simulink model "sampleModel244"  (R2021b)
settings: Solver=VariableStepAuto  StartTime=0.0  StopTime=10.0  RelTol=1e-3
undefined symbols (not defined in the file or in its folder): DiscIntNeverNeededParam
libraries: simulink x13, slpidlib x3
settings Model: Creator=user  LastModifiedBy=user

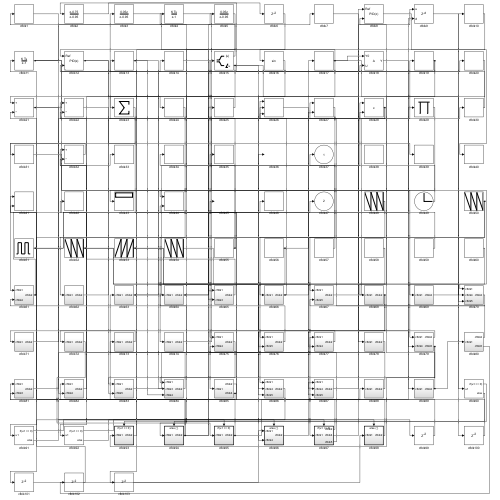
[thumbnail: Simulink's stored preview of the top-level diagram]
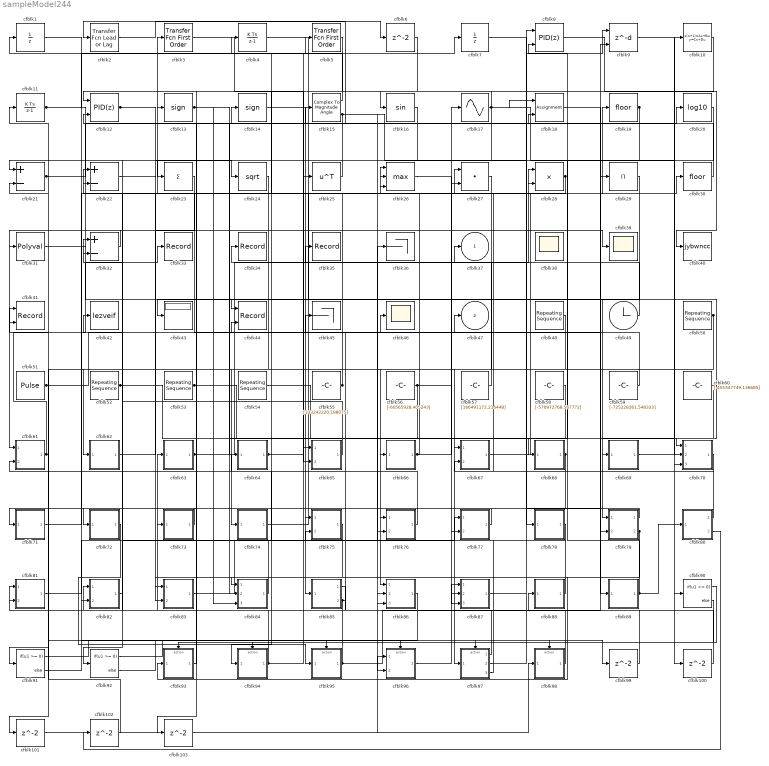
== system sampleModel244 ==
  cfblk1 : UnitDelay  HasFrameUpgradeWarning=on
  cfblk10 : DiscreteStateSpace
  cfblk{6,99..103} (6 alike) : Delay  SampleTime=1
  cfblk11 : DiscreteIntegrator  ICPrevOutput=DiscIntNeverNeededParam  ICPrevScaledInput=DiscIntNeverNeededParam
  cfblk12 : slpidlib/PID Controller (2DOF)  Controller=PID  Form=Parallel  TimeDomain=Discrete-time  UseExternalTs=off  SampleTime=1  IntegratorMethod=Forward Euler  FilterMethod=Forward Euler  ControllerParametersSource=internal  P=1  I=1  D=0  UseFilter=on  N=100  b=1  c=1  TunerSelectOption=Transfer Function Based (PID Tuner App)  InitialConditionSource=internal  InitialConditionForIntegrator=0  InitialConditionForFilter=0  DifferentiatorICPrevScaledInput=0  ExternalReset=none  TrackingMode=off  Kt=1  LimitOutput=off  SatLimitsSource=internal  UpperSaturationLimit=inf  LowerSaturationLimit=-inf  LinearizeAsGain=off  AntiWindupMode=none  Kb=1  POutMin=[]  POutMax=[]  IOutMin=[]  IOutMax=[]  DOutMin=[]  DOutMax=[]  NOutMin=[]  NOutMax=[]  bOutMin=[]  bOutMax=[]  cOutMin=[]  cOutMax=[]  SumOutMin=[]  SumOutMax=[]  SaturationOutMin=[]  SaturationOutMax=[]  PParamMin=[]  PParamMax=[]  IParamMin=[]  IParamMax=[]  DParamMin=[]  DParamMax=[]  NParamMin=[]  NParamMax=[]  bParamMin=[]  bParamMax=[]  cParamMin=[]  cParamMax=[]  KbParamMin=[]  KbParamMax=[]  KtParamMin=[]  KtParamMax=[]  KbOutMin=[]  KbOutMax=[]  KtOutMin=[]  KtOutMax=[]  IntegratorOutMin=[]  IntegratorOutMax=[]  FilterOutMin=[]  FilterOutMax=[]  SumI1OutMin=[]  SumI1OutMax=[]  SumI2OutMin=[]  SumI2OutMax=[]  SumI3OutMin=[]  SumI3OutMax=[]  SumI4OutMin=[]  SumI4OutMax=[]  SumDOutMin=[]  SumDOutMax=[]  Sum1OutMin=[]  Sum1OutMax=[]  Sum2OutMin=[]  Sum2OutMax=[]  Sum3OutMin=[]  Sum3OutMax=[]  DifferentiatorOutMin=[]  DifferentiatorOutMax=[]  FilterDiffOutCoefMin=[]  FilterDiffOutCoefMax=[]  ReciprocalOutMin=[]  ReciprocalOutMax=[]  SumDenOutMin=[]  SumDenOutMax=[]  SumNumOutMin=[]  SumNumOutMax=[]  DivideOutMin=[]  DivideOutMax=[]  UdiffTsProdOutMin=[]  UdiffTsProdOutMax=[]  NTsProdOutMin=[]  NTsProdOutMax=[]  UintegralTsProdOutMin=[]  UintegralTsProdOutMax=[]  UngainTsProdOutMin=[]  UngainTsProdOutMax=[]  IntegratorContinuousStateAttributes=''  IntegratorStateMustResolveToSignalObject=off  IntegratorRTWStateStorageClass=Auto  FilterContinuousStateAttributes=''  FilterStateMustResolveToSignalObject=off  FilterRTWStateStorageClass=Auto  ParallelPVariant=InternalParameters  IdealPVariant=Disabled  IVariant=InternalParameters  DVariant=InternalParameters  bVariant=InternalParameters  cVariant=InternalParameters  IntegratorVariant=Discrete  SatVariant=Disabled  AWVariant=Passthrough  PCopyVariant=Disabled  TRVariant=Disabled  FdbkBlocksVariant=Forward  IdealPFdbkVariant=Disabled  SatFdbkVariant=Disabled  DerivativeFilterVariant=ForwardEulerFilter  NVariant=InternalParameters  NCopyVariant=Disabled  FilterICVariant=InternalICsFilter  IntegratorICVariant=InternalICs  ExternalResetVariant=Disabled  TRSumVariant=Passthrough  SumFdbkVariant=Disabled  SumVariant=Sum_PID  TsampFilterVariant=InternalTs  TsampNgainVariant=Passthrough  TsampIntegralVariant=Passthrough  ExternalSaturationOutDataTypeStr=Inherit: Same as second input
      settings: SourceProductBaseCode=SL
  cfblk13 : Signum
  cfblk14 : Signum
  cfblk15 : ComplexToMagnitudeAngle
  cfblk16 : Trigonometry
  cfblk17 : Sin  TimeSource=Use external signal  SampleTime=0
  cfblk18 : Assignment  DiagnosticForDimensions=Warning  IndexOptions=Index vector (dialog)  Indices=1  OutputSizes=1
  cfblk19 : Rounding
  cfblk2 : simulink/Discrete/Transfer Fcn Lead or Lag  PoleZ=0.95  ZeroZ=0.75  ICPrevOutput=0.0  ICPrevInput=0.0  DoSatur=off
      settings: SourceProductBaseCode=SL
  cfblk20 : Math  Operator=log10  SaturateOnIntegerOverflow=on
  cfblk21 : Sum  Inputs=+-
  cfblk22 : Sum  Inputs=+-
  cfblk23 : Sum  Inputs=+
  cfblk24 : Sqrt  SaturateOnIntegerOverflow=on
  cfblk25 : Math  Operator=transpose  SaturateOnIntegerOverflow=on
  cfblk26 : MinMax  Function=max  Inputs=3
  cfblk27 : DotProduct  InputSameDT=on  OutDataTypeStr=Inherit: Inherit via internal rule
  cfblk28 : Product
  cfblk29 : Product  Inputs=*
  cfblk3 : simulink/Discrete/Transfer Fcn First Order  PoleZ=0.95  ICPrevOutput=0.0  DoSatur=off
  cfblk30 : Rounding
  cfblk31 : Polyval  Coefs=[ +2.081618890e-019, -1.441693666e-014, +4.719686976e-010, -8.536869453e-006, +1.621573104e-001, -8.087801117e+001 ]
  cfblk32 : Sum  Inputs=+-
  cfblk33 : Record  FileSettingsInternal="{\"entries\":[{\"content\":{\"excelSettings\":{\"content\":{},\"type\":\"Streamout.ExcelSettings\"}},\"type\":\"Streamout.FileSettingStorage\",\"uuid\":\"3282f54a-cc87-4849-ac33-639abf907f72\"}],\"packageUris\":[\"http://schema.mathworks.com/mf0/streamout_blocks/R2020a\"],\"version\":\"1.0\"}"  SignalsInternal="{\"entries\":[{\"content\":{\"signals\":[{\"content\":{\"blockPath\":[\"sampleModel244/cfblk33\"],\"channel\":[],\"dimensions\":[1],\"domain\":\"sampleModel244/cfblk33\",\"lineColor\":\"#139fff\",\"plots\":[1],\"port\":1,\"sid\":[\"\"],\"signalID\":9772,\"signalName\":\"cfblk61\"},\"type\":\"RecordBlkView.Signal\",\"uuid\":\"cde80ae1-0f0e-4127-a5a1-a608f97d3de1\"}]},\"type\":\"RecordBlkView.InputSignals\",\"uuid\":\"f8d19e68-2bc8-454d-ba24-e771bdc0d423\"}],\"packageUris\":[\"http://schema.mathworks.com/mf0/streamout_blocks/R2020a\"],\"version\":\"1.0\"}"  VisualizationBindings="{\"sparklinesplugin\":{\"info\":[{\"bindingParametersList\":[],\"subplotID\":1}]}}"
  cfblk34 : Record  FileSettingsInternal="{\"entries\":[{\"content\":{\"excelSettings\":{\"content\":{},\"type\":\"Streamout.ExcelSettings\"}},\"type\":\"Streamout.FileSettingStorage\",\"uuid\":\"1bc6323d-6913-452f-8d92-e743385c7954\"}],\"packageUris\":[\"http://schema.mathworks.com/mf0/streamout_blocks/R2020a\"],\"version\":\"1.0\"}"  SignalsInternal="{\"entries\":[{\"content\":{\"signals\":[{\"content\":{\"blockPath\":[\"sampleModel244/cfblk34\"],\"channel\":[],\"dimensions\":[1],\"domain\":\"sampleModel244/cfblk34\",\"lineColor\":\"#fe330a\",\"plots\":[1],\"port\":1,\"sid\":[\"\"],\"signalID\":9792,\"signalName\":\"cfblk55\"},\"type\":\"RecordBlkView.Signal\",\"uuid\":\"2fd89c6a-0567-430f-a438-ed56d00d60f2\"}]},\"type\":\"RecordBlkView.InputSignals\",\"uuid\":\"daec545a-da82-4114-a5f9-601cc645d5ea\"}],\"packageUris\":[\"http://schema.mathworks.com/mf0/streamout_blocks/R2020a\"],\"version\":\"1.0\"}"  VisualizationBindings="{\"sparklinesplugin\":{\"info\":[{\"bindingParametersList\":[],\"subplotID\":1}]}}"
  cfblk35 : Record  FileSettingsInternal="{\"entries\":[{\"content\":{\"excelSettings\":{\"content\":{},\"type\":\"Streamout.ExcelSettings\"}},\"type\":\"Streamout.FileSettingStorage\",\"uuid\":\"d44ad37f-a161-4993-b71a-48dc8168da26\"}],\"packageUris\":[\"http://schema.mathworks.com/mf0/streamout_blocks/R2020a\"],\"version\":\"1.0\"}"  SignalsInternal="{\"entries\":[{\"content\":{\"signals\":[{\"content\":{\"blockPath\":[\"sampleModel244/cfblk35\"],\"channel\":[],\"dimensions\":[1],\"domain\":\"sampleModel244/cfblk35\",\"lineColor\":\"#22b573\",\"plots\":[1],\"port\":1,\"sid\":[\"\"],\"signalID\":9796,\"signalName\":\"cfblk49\"},\"type\":\"RecordBlkView.Signal\",\"uuid\":\"f63b9365-5ab6-4a57-a3c5-5ba42ee07859\"}]},\"type\":\"RecordBlkView.InputSignals\",\"uuid\":\"8d4ba322-4ce7-4960-87db-79ef0bd083d4\"}],\"packageUris\":[\"http://schema.mathworks.com/mf0/streamout_blocks/R2020a\"],\"version\":\"1.0\"}"  VisualizationBindings="{\"sparklinesplugin\":{\"info\":[{\"bindingParametersList\":[],\"subplotID\":1}]}}"
  cfblk36 : Terminator
  cfblk38 : Scope
      settings: Floating=on
  cfblk39 : Scope
  cfblk4 : DiscreteIntegrator  ICPrevOutput=DiscIntNeverNeededParam  ICPrevScaledInput=DiscIntNeverNeededParam
  cfblk40 : ToWorkspace  VariableName=jybwncc  SaveFormat=Timeseries  SampleTime=-1
  cfblk41 : Record  FileSettingsInternal="{\"entries\":[{\"content\":{\"excelSettings\":{\"content\":{},\"type\":\"Streamout.ExcelSettings\"}},\"type\":\"Streamout.FileSettingStorage\",\"uuid\":\"2a096b76-41e0-4fc9-b8e7-cead69cfeab4\"}],\"packageUris\":[\"http://schema.mathworks.com/mf0/streamout_blocks/R2020a\"],\"version\":\"1.0\"}"  Layout=[1 1]  SignalsInternal="{\"entries\":[{\"content\":{\"signals\":[{\"content\":{\"blockPath\":[\"sampleModel244/cfblk41\"],\"channel\":[],\"dimensions\":[1],\"domain\":\"sampleModel244/cfblk41\",\"lineColor\":\"#a2142f\",\"plots\":[1],\"port\":1,\"sid\":[\"\"],\"signalID\":9776,\"signalName\":\"cfblk76\"},\"type\":\"RecordBlkView.Signal\",\"uuid\":\"448cb670-8667-4582-b93f-e7d89f4c353b\"},{\"content\":{\"blockPath\":[\"sampleModel244/cfblk41\"],\"channel\":[],\"dimensions\":[1],\"domain\":\"sampleModel244/cfblk41\",\"lineColor\":\"#139fff\",\"plots\":[1],\"port\":2,\"sid\":[\"\"],\"signalID\":9780,\"signalName\":\"cfblk95\"},\"type\":\"RecordBlkView.Signal\",\"uuid\":\"49dd1c68-4c2e-4a77-8898-24a62e94df85\"}]},\"type\":\"RecordBlkView.InputSignals\",\"uuid\":\"c0b55ab5-4389-43fe-bc0b-143dab00b9ab\"}],\"packageUris\":[\"http://schema.mathworks.com/mf0/streamout_blocks/R2020a\"],\"version\":\"1.0\"}"  VisualizationBindings="{\"xyplotplugin\":{\"info\":[{\"series\":[{\"bindingParametersList\":[{\"parameter\":\"X-Axis\",\"signalID\":9776,\"signalName\":\"cfblk76\"},{\"parameter\":\"Y-Axis\",\"signalID\":9780,\"signalName\":\"cfblk95\"}],\"seriesID\":58913}],\"subplotID\":1}]}}"  CompatibilityTag=XY
  cfblk42 : ToWorkspace  VariableName=lezveif  SaveFormat=Timeseries  SampleTime=-1
  cfblk43 : Display
  cfblk44 : Record  FileSettingsInternal="{\"entries\":[{\"content\":{\"excelSettings\":{\"content\":{},\"type\":\"Streamout.ExcelSettings\"}},\"type\":\"Streamout.FileSettingStorage\",\"uuid\":\"67c1ab0d-b2bc-48ee-9bb9-5083cd67cfb9\"}],\"packageUris\":[\"http://schema.mathworks.com/mf0/streamout_blocks/R2020a\"],\"version\":\"1.0\"}"  Layout=[1 1]  SignalsInternal="{\"entries\":[{\"content\":{\"signals\":[{\"content\":{\"blockPath\":[\"sampleModel244/cfblk44\"],\"channel\":[],\"dimensions\":[1],\"domain\":\"sampleModel244/cfblk44\",\"lineColor\":\"#a2142f\",\"plots\":[1],\"port\":1,\"sid\":[\"\"],\"signalID\":9784,\"signalName\":\"cfblk16\"},\"type\":\"RecordBlkView.Signal\",\"uuid\":\"b927b068-dea9-4670-ad21-d052ed595eca\"},{\"content\":{\"blockPath\":[\"sampleModel244/cfblk44\"],\"channel\":[],\"dimensions\":[1],\"domain\":\"sampleModel244/cfblk44\",\"lineColor\":\"#139fff\",\"plots\":[1],\"port\":2,\"sid\":[\"\"],\"signalID\":9788,\"signalName\":\"cfblk85:2\"},\"type\":\"RecordBlkView.Signal\",\"uuid\":\"65f9025a-423f-4d0f-be98-834b3f9f0393\"}]},\"type\":\"RecordBlkView.InputSignals\",\"uuid\":\"b847a701-74f3-4d0a-bcda-2eb64e4d33aa\"}],\"packageUris\":[\"http://schema.mathworks.com/mf0/streamout_blocks/R2020a\"],\"version\":\"1.0\"}"  VisualizationBindings="{\"xyplotplugin\":{\"info\":[{\"series\":[{\"bindingParametersList\":[{\"parameter\":\"X-Axis\",\"signalID\":9784,\"signalName\":\"cfblk16\"},{\"parameter\":\"Y-Axis\",\"signalID\":9788,\"signalName\":\"cfblk85:2\"}],\"seriesID\":22887}],\"subplotID\":1}]}}"  CompatibilityTag=XY
  cfblk45 : Terminator
  cfblk46 : Scope
  cfblk48 : simulink/Sources/Repeating Sequence  rep_seq_t=[0 2]  rep_seq_y=[748118952.385065, -429634396.575888]
  cfblk49 : Clock
  cfblk5 : simulink/Discrete/Transfer Fcn First Order  PoleZ=0.95  ICPrevOutput=0.0  DoSatur=off
  cfblk50 : simulink/Sources/Repeating Sequence  rep_seq_t=[0 2]  rep_seq_y=[-7832979.002847, -534327184.207940]
  cfblk51 : DiscretePulseGenerator  PulseType=Time based  Amplitude=[-2375380.359104]  Period=[17929664.950864]  PulseWidth=5  PhaseDelay=[3.000000]
  cfblk52 : simulink/Sources/Repeating Sequence  rep_seq_t=[0 2]  rep_seq_y=[306378667.720082, -357464766.686982]
  cfblk53 : simulink/Sources/Repeating Sequence  rep_seq_t=[0 2]  rep_seq_y=[-57185752.354315, 440238882.703146]
  cfblk54 : simulink/Sources/Repeating Sequence  rep_seq_t=[0 2]  rep_seq_y=[792455784.862972, -745237724.350007]
  cfblk55 : Constant  Value=[333242220.188075]  SampleTime=1
  cfblk56 : Constant  Value=[-60565928.405243]  SampleTime=1
  cfblk57 : Constant  Value=[166491172.216448]  SampleTime=1
  cfblk58 : Constant  Value=[-570972768.567772]  SampleTime=1
  cfblk59 : Constant  Value=[-725228261.548333]  SampleTime=1
  cfblk60 : Constant  Value=[-455347749.136685]  SampleTime=1
  cfblk61 : Subsystem
  cfblk62 : Subsystem
  cfblk63 : Subsystem
  cfblk64 : Subsystem
  cfblk65 : Subsystem
  cfblk66 : Subsystem
  cfblk67 : Subsystem
  cfblk68 : Subsystem
  cfblk69 : Subsystem
  cfblk7 : UnitDelay  HasFrameUpgradeWarning=on
  cfblk70 : Subsystem
  cfblk71 : Subsystem
  cfblk72 : Subsystem
  cfblk73 : Subsystem
  cfblk74 : Subsystem
  cfblk75 : Subsystem
  cfblk76 : Subsystem
  cfblk77 : Subsystem
  cfblk78 : Subsystem
  cfblk79 : Subsystem
  cfblk8 : slpidlib/PID Controller (2DOF)  Controller=PID  Form=Parallel  TimeDomain=Discrete-time  UseExternalTs=off  SampleTime=1  IntegratorMethod=Forward Euler  FilterMethod=Forward Euler  ControllerParametersSource=internal  P=1  I=1  D=0  UseFilter=on  N=100  b=1  c=1  TunerSelectOption=Transfer Function Based (PID Tuner App)  InitialConditionSource=internal  InitialConditionForIntegrator=0  InitialConditionForFilter=0  DifferentiatorICPrevScaledInput=0  ExternalReset=none  TrackingMode=off  Kt=1  LimitOutput=off  SatLimitsSource=internal  UpperSaturationLimit=inf  LowerSaturationLimit=-inf  LinearizeAsGain=off  AntiWindupMode=none  Kb=1  POutMin=[]  POutMax=[]  IOutMin=[]  IOutMax=[]  DOutMin=[]  DOutMax=[]  NOutMin=[]  NOutMax=[]  bOutMin=[]  bOutMax=[]  cOutMin=[]  cOutMax=[]  SumOutMin=[]  SumOutMax=[]  SaturationOutMin=[]  SaturationOutMax=[]  PParamMin=[]  PParamMax=[]  IParamMin=[]  IParamMax=[]  DParamMin=[]  DParamMax=[]  NParamMin=[]  NParamMax=[]  bParamMin=[]  bParamMax=[]  cParamMin=[]  cParamMax=[]  KbParamMin=[]  KbParamMax=[]  KtParamMin=[]  KtParamMax=[]  KbOutMin=[]  KbOutMax=[]  KtOutMin=[]  KtOutMax=[]  IntegratorOutMin=[]  IntegratorOutMax=[]  FilterOutMin=[]  FilterOutMax=[]  SumI1OutMin=[]  SumI1OutMax=[]  SumI2OutMin=[]  SumI2OutMax=[]  SumI3OutMin=[]  SumI3OutMax=[]  SumI4OutMin=[]  SumI4OutMax=[]  SumDOutMin=[]  SumDOutMax=[]  Sum1OutMin=[]  Sum1OutMax=[]  Sum2OutMin=[]  Sum2OutMax=[]  Sum3OutMin=[]  Sum3OutMax=[]  DifferentiatorOutMin=[]  DifferentiatorOutMax=[]  FilterDiffOutCoefMin=[]  FilterDiffOutCoefMax=[]  ReciprocalOutMin=[]  ReciprocalOutMax=[]  SumDenOutMin=[]  SumDenOutMax=[]  SumNumOutMin=[]  SumNumOutMax=[]  DivideOutMin=[]  DivideOutMax=[]  UdiffTsProdOutMin=[]  UdiffTsProdOutMax=[]  NTsProdOutMin=[]  NTsProdOutMax=[]  UintegralTsProdOutMin=[]  UintegralTsProdOutMax=[]  UngainTsProdOutMin=[]  UngainTsProdOutMax=[]  IntegratorContinuousStateAttributes=''  IntegratorStateMustResolveToSignalObject=off  IntegratorRTWStateStorageClass=Auto  FilterContinuousStateAttributes=''  FilterStateMustResolveToSignalObject=off  FilterRTWStateStorageClass=Auto  ParallelPVariant=InternalParameters  IdealPVariant=Disabled  IVariant=InternalParameters  DVariant=InternalParameters  bVariant=InternalParameters  cVariant=InternalParameters  IntegratorVariant=Discrete  SatVariant=Disabled  AWVariant=Passthrough  PCopyVariant=Disabled  TRVariant=Disabled  FdbkBlocksVariant=Forward  IdealPFdbkVariant=Disabled  SatFdbkVariant=Disabled  DerivativeFilterVariant=ForwardEulerFilter  NVariant=InternalParameters  NCopyVariant=Disabled  FilterICVariant=InternalICsFilter  IntegratorICVariant=InternalICs  ExternalResetVariant=Disabled  TRSumVariant=Passthrough  SumFdbkVariant=Disabled  SumVariant=Sum_PID  TsampFilterVariant=InternalTs  TsampNgainVariant=Passthrough  TsampIntegralVariant=Passthrough  ExternalSaturationOutDataTypeStr=Inherit: Same as second input
      settings: SourceProductBaseCode=SL
  cfblk80 : Subsystem
  cfblk81 : Subsystem
  cfblk82 : Subsystem
  cfblk83 : Subsystem
  cfblk84 : Subsystem
  cfblk85 : Subsystem
  cfblk86 : Subsystem
  cfblk87 : Subsystem
  cfblk88 : Subsystem
  cfblk89 : Subsystem
  cfblk9 : Delay  DelayLengthSource=Input port  SampleTime=1
      settings: InputPortMap=u0,p1
  cfblk90 : If  IfExpression=u1 >= 0  SampleTime=1
  cfblk91 : If  IfExpression=u1 >= 0  SampleTime=1
  cfblk92 : If  IfExpression=u1 >= 0  SampleTime=1
  cfblk93 : Subsystem  TreatAsAtomicUnit=on
  cfblk94 : Subsystem  TreatAsAtomicUnit=on
  cfblk95 : Subsystem  TreatAsAtomicUnit=on
  cfblk96 : Subsystem  TreatAsAtomicUnit=on
  cfblk97 : Subsystem  TreatAsAtomicUnit=on
  cfblk98 : Subsystem  TreatAsAtomicUnit=on
  cfblk37 : Outport
  cfblk47 : Outport  Port=2
  wires:
  cfblk50/1 -> cfblk97/1(cfblk1), cfblk91/1
  cfblk4/1 -> cfblk70/1(cfblk1)
  cfblk27/1 -> cfblk86/1(cfblk1)
  cfblk51/1 -> cfblk46/1, cfblk9/2
  cfblk30/1 -> cfblk2/1
  cfblk74/1(cfblk2) -> cfblk30/1
  cfblk57/1 -> cfblk37/1
  cfblk14/1 -> cfblk85/1(cfblk1)
  cfblk85/1(cfblk2) -> cfblk82/1(cfblk1)
  cfblk97/1(cfblk2) -> cfblk63/1(cfblk1)
  cfblk48/1 -> cfblk74/1(cfblk1)
  cfblk61/1(cfblk2) -> cfblk33/1, cfblk21/2
  cfblk66/1(cfblk2) -> cfblk17/1, cfblk26/3
  cfblk73/1(cfblk2) -> cfblk72/1(cfblk1)
  cfblk49/1 -> cfblk35/1
  cfblk79/1(cfblk2) -> cfblk71/1(cfblk1)
  cfblk80/1(cfblk2) -> cfblk27/1
  cfblk15/1 -> cfblk1/1
  cfblk55/1 -> cfblk34/1, cfblk4/1
  cfblk56/1 -> cfblk27/2, cfblk84/2(cfblk3)
  cfblk63/1(cfblk2) -> cfblk28/1, cfblk18/2
  cfblk72/1(cfblk2) -> cfblk95/1(cfblk1)
  cfblk8/1 -> cfblk40/1
  cfblk59/1 -> cfblk3/1
  cfblk83/1(cfblk2) -> cfblk36/1
  cfblk32/1 -> cfblk61/1(cfblk1)
  cfblk82/1(cfblk2) -> cfblk42/1
  cfblk88/1(cfblk2) -> cfblk64/1(cfblk1)
  cfblk79/2(cfblk5) -> cfblk93/1(cfblk1), cfblk84/1(cfblk1)
  cfblk6/1 -> cfblk43/1
  cfblk62/1(cfblk2) -> cfblk28/2
  cfblk67/1(cfblk2) -> cfblk19/1
  cfblk77/1(cfblk2) -> cfblk76/1(cfblk1)
  cfblk76/1(cfblk2) -> cfblk41/1
  cfblk60/1 -> cfblk79/1(cfblk1)
  cfblk21/1 -> cfblk14/1, cfblk99/1
  cfblk3/1 -> cfblk65/1(cfblk1)
  cfblk81/1(cfblk2) -> cfblk77/1(cfblk1)
  cfblk23/1 -> cfblk31/1
  cfblk97/2(cfblk4) -> cfblk8/1
  cfblk20/1 -> cfblk68/1(cfblk1)
  cfblk94/1(cfblk2) -> cfblk25/1, cfblk81/2(cfblk3), cfblk61/2(cfblk4), cfblk20/1
  cfblk31/1 -> cfblk69/1(cfblk1)
  cfblk24/1 -> cfblk62/1(cfblk1)
  cfblk68/1(cfblk2) -> cfblk75/1(cfblk1), cfblk87/3(cfblk5)
  cfblk85/2(cfblk4) -> cfblk81/1(cfblk1), cfblk44/2
  cfblk98/1(cfblk2) -> cfblk45/1
  cfblk18/1 -> cfblk89/1(cfblk1)
  cfblk11/1 -> cfblk77/2(cfblk4), cfblk15/1, cfblk5/1
  cfblk93/1(cfblk2) -> cfblk13/1
  cfblk95/1(cfblk2) -> cfblk29/1, cfblk41/2
  cfblk19/1 -> cfblk23/1, cfblk12/2
  cfblk89/1(cfblk2) -> cfblk8/2, cfblk80/1(cfblk1)
  cfblk7/1 -> cfblk79/2(cfblk4)
  cfblk1/1 -> cfblk82/2(cfblk4)
  cfblk22/1 -> cfblk39/1
  cfblk53/1 -> cfblk67/1(cfblk1), cfblk86/3(cfblk5)
  cfblk69/1(cfblk2) -> cfblk10/1
  cfblk58/1 -> cfblk66/1(cfblk1)
  cfblk84/1(cfblk2) -> cfblk22/1
  cfblk13/1 -> cfblk65/2(cfblk3), cfblk84/3(cfblk4)
  cfblk12/1 -> cfblk83/1(cfblk1), cfblk24/1
  cfblk10/1 -> cfblk94/1(cfblk1)
  cfblk52/1 -> cfblk70/2(cfblk4), cfblk76/2(cfblk5)
  cfblk2/1 -> cfblk6/1
  cfblk65/1(cfblk2) -> cfblk32/1
  cfblk5/1 -> cfblk12/1
  cfblk15/2 -> cfblk96/2(cfblk4), cfblk92/1, cfblk78/1(cfblk1)
  cfblk26/1 -> cfblk87/2(cfblk4)
  cfblk71/1(cfblk2) -> cfblk26/1
  cfblk54/1 -> cfblk70/3(cfblk5)
  cfblk17/1 -> cfblk90/1, cfblk18/1, cfblk86/2(cfblk4), cfblk16/1
  cfblk96/1(cfblk2) -> cfblk88/1(cfblk1)
  cfblk28/1 -> cfblk22/2, cfblk26/2
  cfblk87/1(cfblk2) -> cfblk9/1
  cfblk64/1(cfblk2) -> cfblk47/1, cfblk7/1
  cfblk70/1(cfblk2) -> cfblk67/2(cfblk5)
  cfblk16/1 -> cfblk44/1
  cfblk78/1(cfblk2) -> cfblk75/2(cfblk4)
  cfblk75/1(cfblk2) -> cfblk83/2(cfblk5)
  cfblk25/1 -> cfblk21/1
  cfblk97/3(cfblk5) -> cfblk73/1(cfblk1)
  cfblk90/1 -> cfblk93/Action
  cfblk90/2 -> cfblk94/Action
  cfblk91/1 -> cfblk95/Action
  cfblk91/2 -> cfblk96/Action
  cfblk92/1 -> cfblk97/Action
  cfblk92/2 -> cfblk98/Action
  cfblk99/1 -> cfblk32/2
  cfblk9/1 -> cfblk100/1
  cfblk100/1 -> cfblk87/1(cfblk1)
  cfblk86/1(cfblk2) -> cfblk101/1
  cfblk101/1 -> cfblk98/1(cfblk1)
  cfblk80/2(cfblk5) -> cfblk102/1
  cfblk102/1 -> cfblk11/1
  cfblk29/1 -> cfblk103/1
  cfblk103/1 -> cfblk96/1(cfblk1)

== system sampleModel244/cfblk61 ==
  cfblk1 : Inport
  cfblk4 : Inport  Port=2
  cfblk3 : Sqrt  SaturateOnIntegerOverflow=on
  cfblk2 : Outport
  wires:
  cfblk4/1 -> cfblk2/1
  cfblk1/1 -> cfblk3/1

== system sampleModel244/cfblk62 ==
  cfblk1 : Inport
  cfblk3 : Constant  Value=[471527831.339368]  SampleTime=1
  cfblk2 : Outport
  wires:
  cfblk1/1 -> cfblk2/1

== system sampleModel244/cfblk63 ==
  cfblk1 : Inport
  cfblk3 : Constant  Value=[266532891.050368]  SampleTime=1
  cfblk4 : Constant  Value=[-461865537.627971]  SampleTime=1
  cfblk2 : Outport
  wires:
  cfblk4/1 -> cfblk2/1

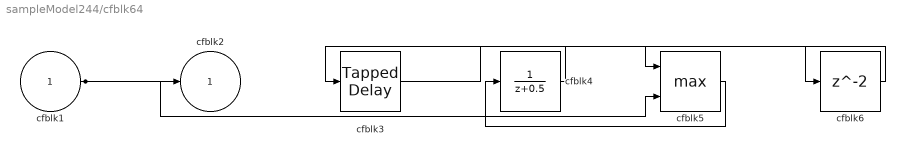
== system sampleModel244/cfblk64 ==
  cfblk1 : Inport
  cfblk3 : simulink/Discrete/Tapped Delay  vinit=0.0  samptime=-1  NumDelays=1  DelayOrder=Oldest  includeCurrent=off
  cfblk4 : DiscreteTransferFcn  SampleTime=1
  cfblk5 : MinMax  Function=max  Inputs=2
  cfblk6 : Delay  SampleTime=1
  cfblk2 : Outport
  wires:
  cfblk4/1 -> cfblk3/1
  cfblk1/1 -> cfblk2/1, cfblk5/2
  cfblk5/1 -> cfblk4/1
  cfblk3/1 -> cfblk6/1
  cfblk6/1 -> cfblk5/1

== system sampleModel244/cfblk65 ==
  cfblk1 : Inport
  cfblk3 : Inport  Port=2
  cfblk2 : Outport
  wires:
  cfblk3/1 -> cfblk2/1

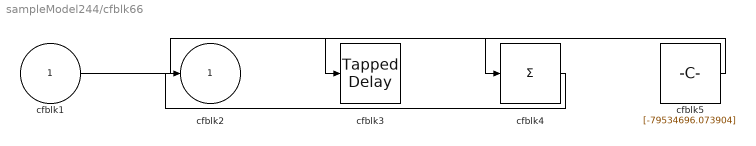
== system sampleModel244/cfblk66 ==
  cfblk1 : Inport
  cfblk3 : simulink/Discrete/Tapped Delay  vinit=0.0  samptime=-1  NumDelays=1  DelayOrder=Oldest  includeCurrent=off
  cfblk4 : Sum  Inputs=+
  cfblk5 : Constant  Value=[-79534696.073904]  SampleTime=1
  cfblk2 : Outport
  wires:
  cfblk1/1 -> cfblk4/1
  cfblk4/1 -> cfblk2/1
  cfblk5/1 -> cfblk3/1

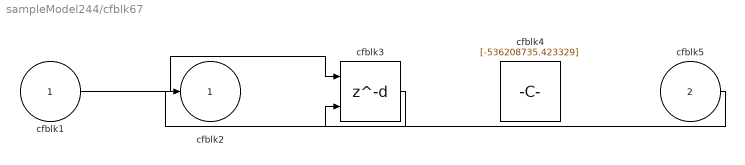
== system sampleModel244/cfblk67 ==
  cfblk1 : Inport
  cfblk5 : Inport  Port=2
  cfblk3 : Delay  DelayLengthSource=Input port  SampleTime=1
      settings: InputPortMap=u0,p1
  cfblk4 : Constant  Value=[-536208735.423329]  SampleTime=1
  cfblk2 : Outport
  wires:
  cfblk1/1 -> cfblk3/1
  cfblk3/1 -> cfblk2/1
  cfblk5/1 -> cfblk3/2

== system sampleModel244/cfblk68 ==
  cfblk1 : Inport
  cfblk3 : Sum  Inputs=+-
  cfblk2 : Outport
  wires:
  cfblk1/1 -> cfblk2/1, cfblk3/1, cfblk3/2

== system sampleModel244/cfblk69 ==
  cfblk1 : Inport
  cfblk3 : DiscreteStateSpace
  cfblk4 : DiscreteTransferFcn  SampleTime=1
  cfblk2 : Outport
  wires:
  cfblk4/1 -> cfblk3/1
  cfblk1/1 -> cfblk4/1
  cfblk3/1 -> cfblk2/1

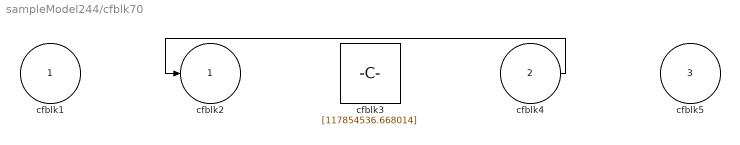
== system sampleModel244/cfblk70 ==
  cfblk1 : Inport
  cfblk4 : Inport  Port=2
  cfblk5 : Inport  Port=3
  cfblk3 : Constant  Value=[117854536.668014]  SampleTime=1
  cfblk2 : Outport
  wires:
  cfblk4/1 -> cfblk2/1

== system sampleModel244/cfblk71 ==
  cfblk1 : Inport
  cfblk3 : Bias  Bias=[712286684.811719]
  cfblk2 : Outport
  wires:
  cfblk1/1 -> cfblk3/1
  cfblk3/1 -> cfblk2/1

== system sampleModel244/cfblk72 ==
  cfblk1 : Inport
  cfblk3 : Reshape
  cfblk2 : Outport
  wires:
  cfblk1/1 -> cfblk2/1, cfblk3/1

== system sampleModel244/cfblk73 ==
  cfblk1 : Inport
  cfblk3 : simulink/Math Operations/MinMax Running Resettable  Function=min  vinit=0.0
  cfblk2 : Outport
  wires:
  cfblk1/1 -> cfblk2/1, cfblk3/1, cfblk3/2

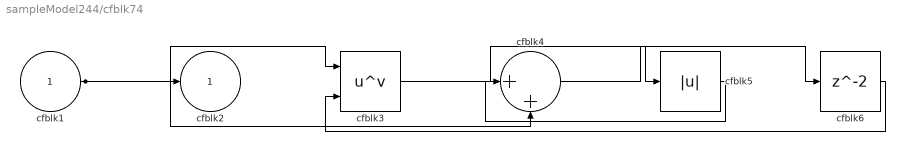
== system sampleModel244/cfblk74 ==
  cfblk1 : Inport
  cfblk3 : Math  Operator=pow  SaturateOnIntegerOverflow=on
  cfblk4 : Sum  Inputs=|++
  cfblk5 : Abs
  cfblk6 : Delay  SampleTime=1
  cfblk2 : Outport
  wires:
  cfblk1/1 -> cfblk3/1, cfblk4/2, cfblk2/1
  cfblk3/1 -> cfblk5/1
  cfblk5/1 -> cfblk4/1
  cfblk4/1 -> cfblk6/1
  cfblk6/1 -> cfblk3/2

== system sampleModel244/cfblk75 ==
  cfblk1 : Inport
  cfblk4 : Inport  Port=2
  cfblk3 : Sum  Inputs=+-
  cfblk2 : Outport
  wires:
  cfblk1/1 -> cfblk3/1
  cfblk3/1 -> cfblk2/1
  cfblk4/1 -> cfblk3/2

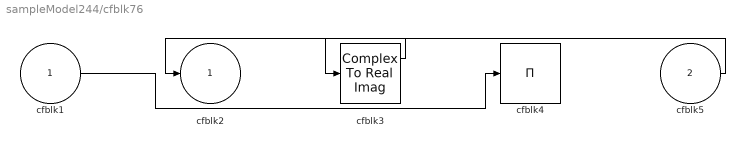
== system sampleModel244/cfblk76 ==
  cfblk1 : Inport
  cfblk5 : Inport  Port=2
  cfblk3 : ComplexToRealImag
  cfblk4 : Product  Inputs=*
  cfblk2 : Outport
  wires:
  cfblk3/1 -> cfblk2/1
  cfblk1/1 -> cfblk4/1
  cfblk5/1 -> cfblk3/1

== system sampleModel244/cfblk77 ==
  cfblk1 : Inport
  cfblk4 : Inport  Port=2
  cfblk3 : DotProduct  InputSameDT=on  OutDataTypeStr=Inherit: Inherit via internal rule
  cfblk2 : Outport
  wires:
  cfblk4/1 -> cfblk3/1
  cfblk1/1 -> cfblk3/2
  cfblk3/1 -> cfblk2/1

== system sampleModel244/cfblk78 ==
  cfblk1 : Inport
  cfblk3 : DiscreteFir  SampleTime=1
  cfblk2 : Outport
  wires:
  cfblk1/1 -> cfblk3/1
  cfblk3/1 -> cfblk2/1

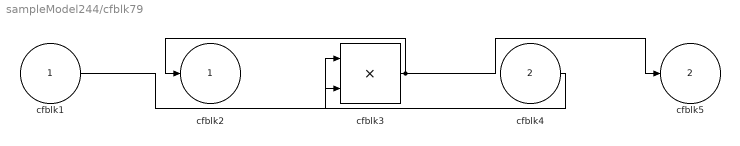
== system sampleModel244/cfblk79 ==
  cfblk1 : Inport
  cfblk4 : Inport  Port=2
  cfblk3 : Product
  cfblk2 : Outport
  cfblk5 : Outport  Port=2
  wires:
  cfblk3/1 -> cfblk2/1, cfblk5/1
  cfblk1/1 -> cfblk3/1
  cfblk4/1 -> cfblk3/2

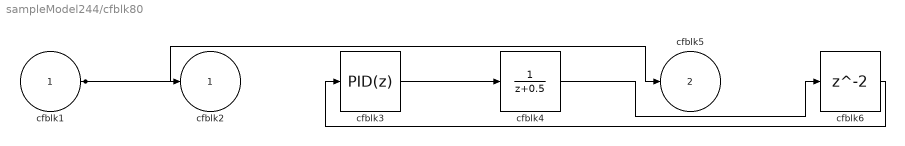
== system sampleModel244/cfblk80 ==
  cfblk1 : Inport
  cfblk3 : slpidlib/PID Controller  Controller=PID  Form=Parallel  TimeDomain=Discrete-time  UseExternalTs=off  SampleTime=1  IntegratorMethod=Forward Euler  FilterMethod=Forward Euler  ControllerParametersSource=internal  P=1  I=1  D=0  UseFilter=on  N=100  TunerSelectOption=Transfer Function Based (PID Tuner App)  InitialConditionSource=internal  InitialConditionForIntegrator=0  InitialConditionForFilter=0  DifferentiatorICPrevScaledInput=0  ExternalReset=none  TrackingMode=off  Kt=1  LimitOutput=off  SatLimitsSource=internal  UpperSaturationLimit=inf  LowerSaturationLimit=-inf  LinearizeAsGain=off  AntiWindupMode=none  Kb=1  POutMin=[]  POutMax=[]  IOutMin=[]  IOutMax=[]  DOutMin=[]  DOutMax=[]  NOutMin=[]  NOutMax=[]  SumOutMin=[]  SumOutMax=[]  SaturationOutMin=[]  SaturationOutMax=[]  PParamMin=[]  PParamMax=[]  IParamMin=[]  IParamMax=[]  DParamMin=[]  DParamMax=[]  NParamMin=[]  NParamMax=[]  KbParamMin=[]  KbParamMax=[]  KtParamMin=[]  KtParamMax=[]  KbOutMin=[]  KbOutMax=[]  KtOutMin=[]  KtOutMax=[]  IntegratorOutMin=[]  IntegratorOutMax=[]  FilterOutMin=[]  FilterOutMax=[]  SumI1OutMin=[]  SumI1OutMax=[]  SumI2OutMin=[]  SumI2OutMax=[]  SumI3OutMin=[]  SumI3OutMax=[]  SumI4OutMin=[]  SumI4OutMax=[]  SumDOutMin=[]  SumDOutMax=[]  DifferentiatorOutMin=[]  DifferentiatorOutMax=[]  FilterDiffOutCoefMin=[]  FilterDiffOutCoefMax=[]  ReciprocalOutMin=[]  ReciprocalOutMax=[]  SumDenOutMin=[]  SumDenOutMax=[]  SumNumOutMin=[]  SumNumOutMax=[]  DivideOutMin=[]  DivideOutMax=[]  UdiffTsProdOutMin=[]  UdiffTsProdOutMax=[]  NTsProdOutMin=[]  NTsProdOutMax=[]  UintegralTsProdOutMin=[]  UintegralTsProdOutMax=[]  UngainTsProdOutMin=[]  UngainTsProdOutMax=[]  IntegratorContinuousStateAttributes=''  IntegratorStateMustResolveToSignalObject=off  IntegratorRTWStateStorageClass=Auto  FilterContinuousStateAttributes=''  FilterStateMustResolveToSignalObject=off  FilterRTWStateStorageClass=Auto  ParallelPVariant=InternalParameters  IdealPVariant=Disabled  IVariant=InternalParameters  DVariant=InternalParameters  IntegratorVariant=Discrete  SatVariant=Disabled  AWVariant=Passthrough  PCopyVariant=Disabled  TRVariant=Disabled  FdbkBlocksVariant=Forward  IdealPFdbkVariant=Disabled  SatFdbkVariant=Disabled  DerivativeFilterVariant=ForwardEulerFilter  NVariant=InternalParameters  NCopyVariant=Disabled  FilterICVariant=InternalICsFilter  IntegratorICVariant=InternalICs  ExternalResetVariant=Disabled  TRSumVariant=Passthrough  SumFdbkVariant=Disabled  SumVariant=Sum_PID  TsampFilterVariant=InternalTs  TsampNgainVariant=Passthrough  TsampIntegralVariant=Passthrough  ExternalSaturationOutDataTypeStr=Inherit: Same as second input
  cfblk4 : DiscreteTransferFcn  SampleTime=1
  cfblk6 : Delay  SampleTime=1
  cfblk2 : Outport
  cfblk5 : Outport  Port=2
  wires:
  cfblk1/1 -> cfblk5/1, cfblk2/1
  cfblk3/1 -> cfblk4/1
  cfblk4/1 -> cfblk6/1
  cfblk6/1 -> cfblk3/1

== system sampleModel244/cfblk81 ==
  cfblk1 : Inport
  cfblk3 : Inport  Port=2
  cfblk2 : Outport
  wires:
  cfblk3/1 -> cfblk2/1

== system sampleModel244/cfblk82 ==
  cfblk1 : Inport
  cfblk4 : Inport  Port=2
  cfblk3 : Bias  Bias=[71432375.219163]
  cfblk2 : Outport
  wires:
  cfblk3/1 -> cfblk2/1
  cfblk1/1 -> cfblk3/1

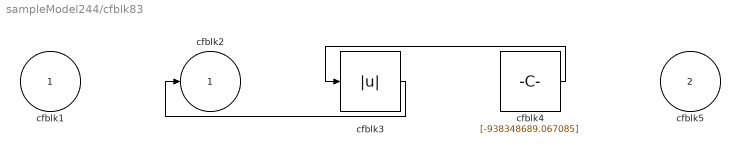
== system sampleModel244/cfblk83 ==
  cfblk1 : Inport
  cfblk5 : Inport  Port=2
  cfblk3 : Abs
  cfblk4 : Constant  Value=[-938348689.067085]  SampleTime=1
  cfblk2 : Outport
  wires:
  cfblk4/1 -> cfblk3/1
  cfblk3/1 -> cfblk2/1

== system sampleModel244/cfblk84 ==
  cfblk1 : Inport
  cfblk3 : Inport  Port=2
  cfblk4 : Inport  Port=3
  cfblk2 : Outport
  wires:
  cfblk4/1 -> cfblk2/1

== system sampleModel244/cfblk85 ==
  cfblk1 : Inport
  cfblk3 : simulink/Discrete/Transfer Fcn Lead or Lag  PoleZ=0.95  ZeroZ=0.75  ICPrevOutput=0.0  ICPrevInput=0.0  DoSatur=off
      settings: SourceProductBaseCode=SL
  cfblk2 : Outport
  cfblk4 : Outport  Port=2
  wires:
  cfblk3/1 -> cfblk4/1
  cfblk1/1 -> cfblk2/1, cfblk3/1

== system sampleModel244/cfblk86 ==
  cfblk1 : Inport
  cfblk4 : Inport  Port=2
  cfblk5 : Inport  Port=3
  cfblk3 : Constant  Value=[-240087962.426565]  SampleTime=1
  cfblk2 : Outport
  wires:
  cfblk5/1 -> cfblk2/1

== system sampleModel244/cfblk87 ==
  cfblk1 : Inport
  cfblk4 : Inport  Port=2
  cfblk5 : Inport  Port=3
  cfblk3 : Trigonometry
  cfblk2 : Outport
  wires:
  cfblk3/1 -> cfblk2/1
  cfblk1/1 -> cfblk3/1

== system sampleModel244/cfblk88 ==
  cfblk1 : Inport
  cfblk3 : Sin  TimeSource=Use external signal  SampleTime=0
  cfblk4 : Trigonometry
  cfblk5 : Delay  SampleTime=1
  cfblk2 : Outport
  wires:
  cfblk1/1 -> cfblk2/1
  cfblk3/1 -> cfblk4/1
  cfblk4/1 -> cfblk5/1
  cfblk5/1 -> cfblk3/1

== system sampleModel244/cfblk89 ==
  cfblk1 : Inport
  cfblk3 : Sqrt  SaturateOnIntegerOverflow=on
  cfblk4 : Gain  Gain=[-102530974.269813]
  cfblk5 : Delay  SampleTime=1
  cfblk2 : Outport
  wires:
  cfblk3/1 -> cfblk4/1
  cfblk1/1 -> cfblk2/1
  cfblk4/1 -> cfblk5/1
  cfblk5/1 -> cfblk3/1

== system sampleModel244/cfblk93 ==
  cfblk1 : Inport
  Action Port : ActionPort  ActionPortLabel=if(u1 >= 0)
  cfblk3 : Sum  Inputs=+
  cfblk2 : Outport
  wires:
  cfblk3/1 -> cfblk2/1
  cfblk1/1 -> cfblk3/1

== system sampleModel244/cfblk94 ==
  cfblk1 : Inport
  Action Port : ActionPort  ActionPortLabel=else
  cfblk3 : Bias  Bias=[993076824.552580]
  cfblk2 : Outport
  wires:
  cfblk1/1 -> cfblk3/1
  cfblk3/1 -> cfblk2/1

== system sampleModel244/cfblk95 ==
  cfblk1 : Inport
  Action Port : ActionPort  ActionPortLabel=if(u1 >= 0)
  cfblk3 : DiscreteStateSpace  SampleTime=-1
  cfblk4 : simulink/Discrete/Difference  ICPrevInput=0.0  OutMin=[]  OutMax=[]  OutDataTypeStr=Inherit: Inherit via back propagation  OutDataType=fixdt(1, 16)  OutScaling=2^-10  DoSatur=off
  cfblk2 : Outport
  wires:
  cfblk4/1 -> cfblk2/1
  cfblk1/1 -> cfblk3/1
  cfblk3/1 -> cfblk4/1

== system sampleModel244/cfblk96 ==
  cfblk1 : Inport
  cfblk4 : Inport  Port=2
  Action Port : ActionPort  ActionPortLabel=else
  cfblk3 : Sum  Inputs=|++
  cfblk2 : Outport
  wires:
  cfblk1/1 -> cfblk2/1, cfblk3/2
  cfblk4/1 -> cfblk3/1

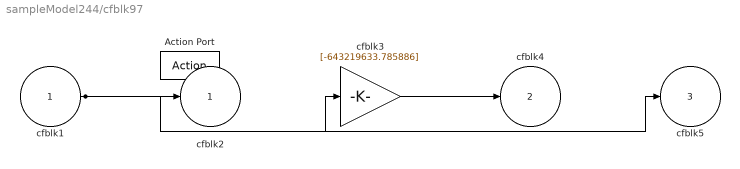
== system sampleModel244/cfblk97 ==
  cfblk1 : Inport
  Action Port : ActionPort  ActionPortLabel=if(u1 >= 0)
  cfblk3 : Gain  Gain=[-643219633.785886]
  cfblk2 : Outport
  cfblk4 : Outport  Port=2
  cfblk5 : Outport  Port=3
  wires:
  cfblk3/1 -> cfblk4/1
  cfblk1/1 -> cfblk2/1, cfblk3/1, cfblk5/1

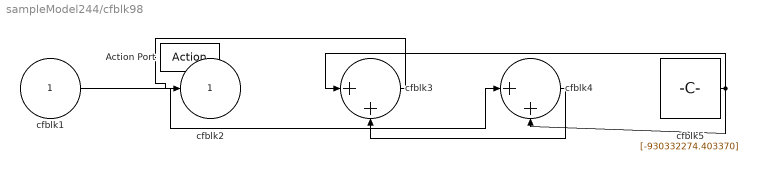
== system sampleModel244/cfblk98 ==
  cfblk1 : Inport
  Action Port : ActionPort  ActionPortLabel=else
  cfblk3 : Sum  Inputs=|++
  cfblk4 : Sum  Inputs=|++
  cfblk5 : Constant  Value=[-930332274.403370]  SampleTime=1
  cfblk2 : Outport
  wires:
  cfblk1/1 -> cfblk4/1
  cfblk3/1 -> cfblk2/1
  cfblk5/1 -> cfblk3/1, cfblk4/2
  cfblk4/1 -> cfblk3/2
